simulink model "final_seatmodel_2_version19a"  (R2019a)
settings: Solver=FixedStepAuto  StartTime=0.0  StopTime=50  FixedStep=1  RelTol=1e-3
undefined symbols (not defined in the file or in its folder): F_B_Motion, Head_Rest, Seat_Height, Seat_Recline, Thai_Support
libraries: powerlib_meascontrol x10, simulink x10
settings Model: Creator=A  LastModifiedBy=A

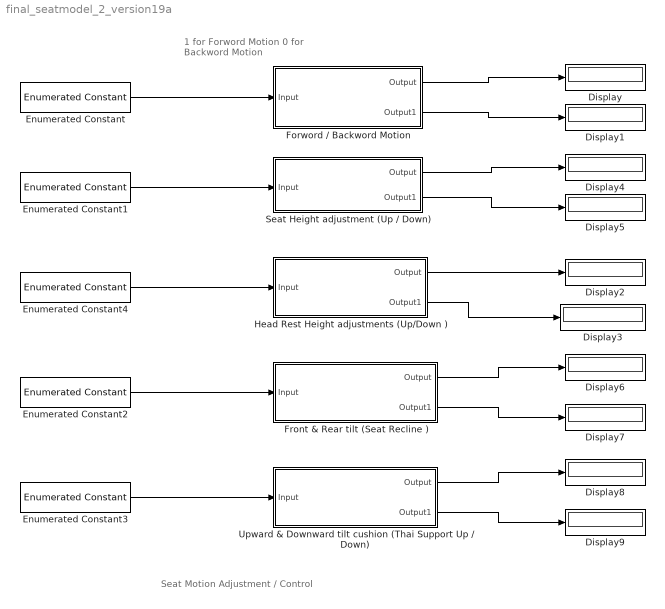
== system final_seatmodel_2_version19a ==
  note: Seat Motion Adjustment / Control
  note: 1 for Forword Motion
      | 0 for Backword Motion
  " Upward & Downward tilt cushion (Thai Support Up / Down) " : Subsystem
  Display{,1..9} (10 alike) : Display
  Enumerated Constant : simulink/Sources/Enumerated Constant  OutDataTypeStr=Enum:F_B_Motion  Value=F_B_Motion.Backword  SampleTime=inf
  Enumerated Constant1 : simulink/Sources/Enumerated Constant  OutDataTypeStr=Enum:Seat_Height  Value=Seat_Height.Down  SampleTime=inf
  Enumerated Constant2 : simulink/Sources/Enumerated Constant  OutDataTypeStr=Enum:Seat_Recline  Value=Seat_Recline.Backword  SampleTime=inf
  Enumerated Constant3 : simulink/Sources/Enumerated Constant  OutDataTypeStr=Enum:Thai_Support  Value=Thai_Support.Down  SampleTime=inf
  Enumerated Constant4 : simulink/Sources/Enumerated Constant  OutDataTypeStr=Enum:Head_Rest  Value=Head_Rest.Down  SampleTime=inf
  Forword / Backword Motion : Subsystem
  "Front & Rear tilt (Seat Recline ) " : Subsystem
  "Head Rest Height adjustments (Up/Down ) " : Subsystem
  "Seat Height adjustment (Up / Down) " : Subsystem
  wires:
  Enumerated Constant3/1 -> " Upward & Downward tilt cushion (Thai Support Up / Down) "/1(Input)
  " Upward & Downward tilt cushion (Thai Support Up / Down) "/1(Output) -> Display8/1
  " Upward & Downward tilt cushion (Thai Support Up / Down) "/2(Output1) -> Display9/1
  Enumerated Constant2/1 -> "Front & Rear tilt (Seat Recline ) "/1(Input)
  "Front & Rear tilt (Seat Recline ) "/1(Output) -> Display6/1
  "Front & Rear tilt (Seat Recline ) "/2(Output1) -> Display7/1
  Enumerated Constant/1 -> Forword / Backword Motion/1(Input)
  Enumerated Constant1/1 -> "Seat Height adjustment (Up / Down) "/1(Input)
  "Seat Height adjustment (Up / Down) "/1(Output) -> Display4/1
  "Seat Height adjustment (Up / Down) "/2(Output1) -> Display5/1
  Enumerated Constant4/1 -> "Head Rest Height adjustments (Up/Down ) "/1(Input)
  "Head Rest Height adjustments (Up/Down ) "/1(Output) -> Display2/1
  "Head Rest Height adjustments (Up/Down ) "/2(Output1) -> Display3/1
  Forword / Backword Motion/2(Output1) -> Display1/1
  Forword / Backword Motion/1(Output) -> Display/1

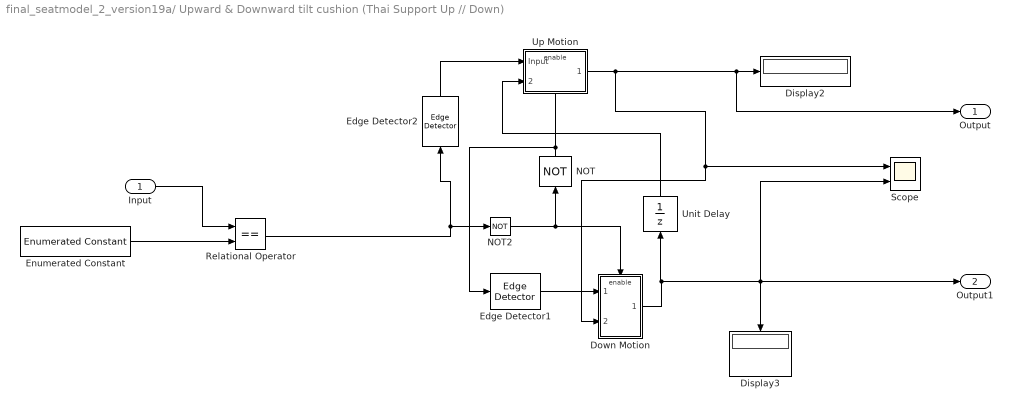
== system final_seatmodel_2_version19a/ Upward & Downward tilt cushion (Thai Support Up // Down)  ==
  Input : Inport
  Display2 : Display
  Display3 : Display
  Down Motion : Subsystem
  Edge Detector1 : powerlib_meascontrol/Logic/Edge Detector  model=Falling  ic=1  Ts=0
      settings: SourceProductBaseCode=PS
  Edge Detector2 : powerlib_meascontrol/Logic/Edge Detector  model=Rising  ic=1  Ts=0
      settings: SourceProductBaseCode=PS
  Enumerated Constant : simulink/Sources/Enumerated Constant  OutDataTypeStr=Enum:Thai_Support  Value=Thai_Support.Up  SampleTime=inf
  NOT : Logic  Operator=NOT  IconShape=distinctive  AllPortsSameDT=off  OutDataTypeStr=boolean
  NOT2 : Logic  Operator=NOT  IconShape=distinctive  AllPortsSameDT=off  OutDataTypeStr=boolean
  Relational Operator : RelationalOperator  Operator===  OutDataTypeStr=boolean  RndMeth=Simplest
  Scope : Scope  NumInputPorts=2
  Unit Delay : UnitDelay  SampleTime=-1  HasFrameUpgradeWarning=on
  Up Motion : Subsystem
  Output : Outport
  Output1 : Outport  Port=2
  wires:
  NOT/1 -> Edge Detector1/1, Up Motion/Enable
  Edge Detector1/1 -> Down Motion/1(Input)
  Down Motion/1(Output) -> Unit Delay/1, Output1/1, Display3/1, Scope/2
  Edge Detector2/1 -> Up Motion/1(Input)
  Relational Operator/1 -> Edge Detector2/1, NOT2/1
  Up Motion/1(Output1) -> Down Motion/2(Input1), Scope/1, Output/1, Display2/1
  Unit Delay/1 -> Up Motion/2(Input1)
  NOT2/1 -> Down Motion/Enable, NOT/1
  Enumerated Constant/1 -> Relational Operator/2
  Input/1 -> Relational Operator/1

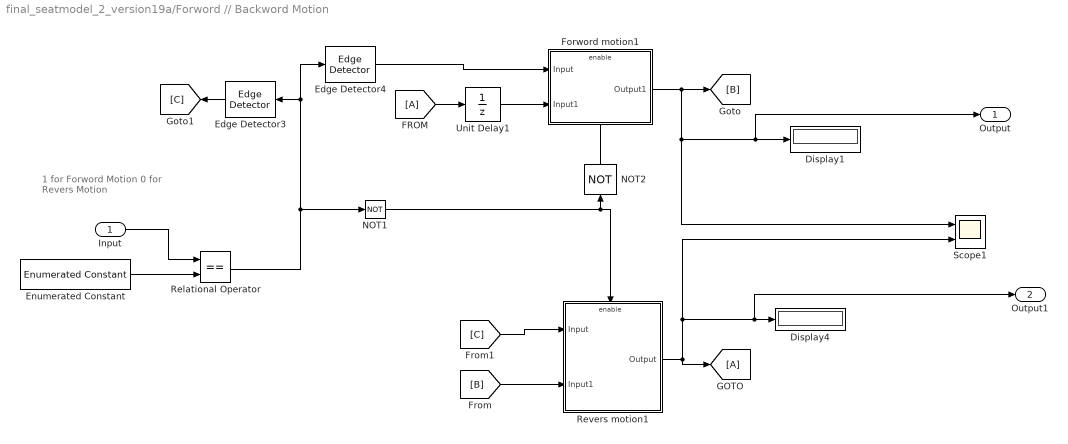
== system final_seatmodel_2_version19a/Forword // Backword Motion ==
  note: 1 for Forword Motion
      | 0 for Revers Motion
  Input : Inport
  Display1 : Display
  Display4 : Display
  Edge Detector3 : powerlib_meascontrol/Logic/Edge Detector  model=Falling  ic=1  Ts=0
      settings: SourceProductBaseCode=PS
  Edge Detector4 : powerlib_meascontrol/Logic/Edge Detector  model=Rising  ic=1  Ts=0
      settings: SourceProductBaseCode=PS
  Enumerated Constant : simulink/Sources/Enumerated Constant  OutDataTypeStr=Enum:F_B_Motion  Value=F_B_Motion.Forword  SampleTime=inf
  Forword motion1 : Subsystem
  NOT1 : Logic  Operator=NOT  IconShape=distinctive  AllPortsSameDT=off  OutDataTypeStr=boolean
  NOT2 : Logic  Operator=NOT  IconShape=distinctive  AllPortsSameDT=off  OutDataTypeStr=boolean
  Relational Operator : RelationalOperator  Operator===  OutDataTypeStr=boolean  RndMeth=Simplest
  Revers motion1 : Subsystem
  Scope1 : Scope  NumInputPorts=2
  Unit Delay1 : UnitDelay  SampleTime=-1  HasFrameUpgradeWarning=on
  Output : Outport
  Output1 : Outport  Port=2
  wires:
  Forword motion1/1(Output1) -> Output/1, Display1/1, Scope1/1, [B]
  Edge Detector3/1 -> [C]
  Revers motion1/1(Output) -> [A], Output1/1, Display4/1, Scope1/2
  Relational Operator/1 -> Edge Detector3/1, Edge Detector4/1, NOT1/1
  NOT2/1 -> Forword motion1/Enable
  [A] -> Unit Delay1/1
  Unit Delay1/1 -> Forword motion1/2(Input1)
  [B] -> Revers motion1/2(Input1)
  Edge Detector4/1 -> Forword motion1/1(Input)
  [C] -> Revers motion1/1(Input)
  NOT1/1 -> Revers motion1/Enable, NOT2/1
  Enumerated Constant/1 -> Relational Operator/2
  Input/1 -> Relational Operator/1

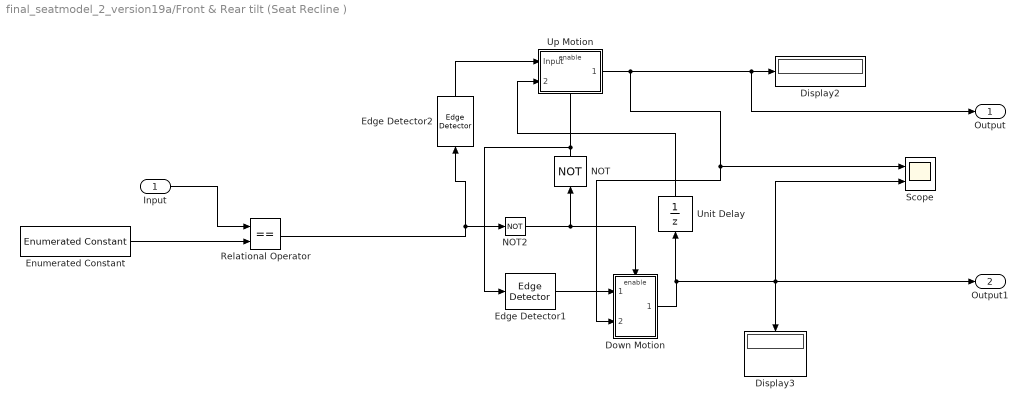
== system final_seatmodel_2_version19a/Front & Rear tilt (Seat Recline )  ==
  Input : Inport
  Display2 : Display
  Display3 : Display
  Down Motion : Subsystem
  Edge Detector1 : powerlib_meascontrol/Logic/Edge Detector  model=Falling  ic=1  Ts=0
      settings: SourceProductBaseCode=PS
  Edge Detector2 : powerlib_meascontrol/Logic/Edge Detector  model=Rising  ic=1  Ts=0
      settings: SourceProductBaseCode=PS
  Enumerated Constant : simulink/Sources/Enumerated Constant  OutDataTypeStr=Enum:Seat_Recline  Value=Seat_Recline.Forword  SampleTime=inf
  NOT : Logic  Operator=NOT  IconShape=distinctive  AllPortsSameDT=off  OutDataTypeStr=boolean
  NOT2 : Logic  Operator=NOT  IconShape=distinctive  AllPortsSameDT=off  OutDataTypeStr=boolean
  Relational Operator : RelationalOperator  Operator===  OutDataTypeStr=boolean  RndMeth=Simplest
  Scope : Scope  NumInputPorts=2
  Unit Delay : UnitDelay  SampleTime=-1  HasFrameUpgradeWarning=on
  Up Motion : Subsystem
  Output : Outport
  Output1 : Outport  Port=2
  wires:
  NOT/1 -> Edge Detector1/1, Up Motion/Enable
  Edge Detector1/1 -> Down Motion/1(Input)
  Down Motion/1(Output) -> Unit Delay/1, Output1/1, Display3/1, Scope/2
  Edge Detector2/1 -> Up Motion/1(Input)
  Relational Operator/1 -> Edge Detector2/1, NOT2/1
  Up Motion/1(Output1) -> Down Motion/2(Input1), Scope/1, Output/1, Display2/1
  Unit Delay/1 -> Up Motion/2(Input1)
  NOT2/1 -> Down Motion/Enable, NOT/1
  Enumerated Constant/1 -> Relational Operator/2
  Input/1 -> Relational Operator/1

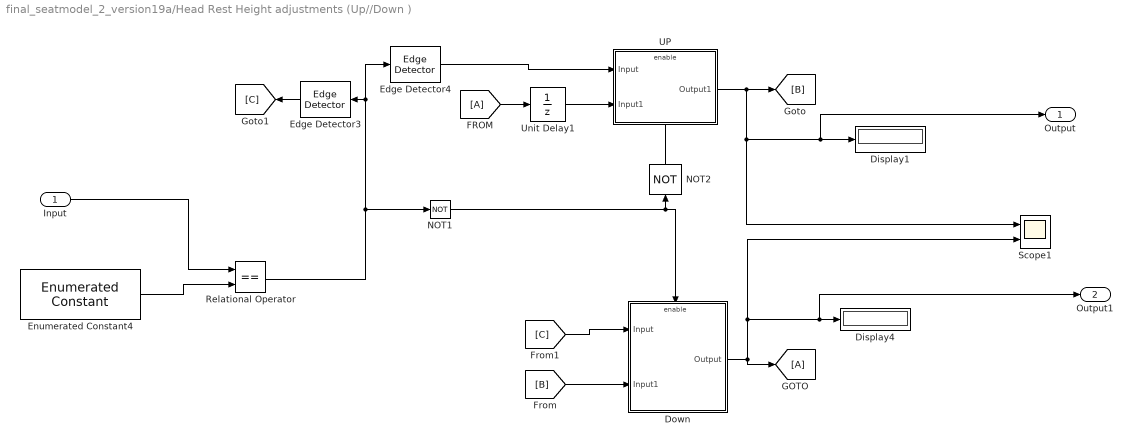
== system final_seatmodel_2_version19a/Head Rest Height adjustments (Up//Down )  ==
  Input : Inport
  Display1 : Display
  Display4 : Display
  Down : Subsystem
  Edge Detector3 : powerlib_meascontrol/Logic/Edge Detector  model=Falling  ic=1  Ts=0
      settings: SourceProductBaseCode=PS
  Edge Detector4 : powerlib_meascontrol/Logic/Edge Detector  model=Rising  ic=1  Ts=0
      settings: SourceProductBaseCode=PS
  Enumerated Constant4 : simulink/Sources/Enumerated Constant  OutDataTypeStr=Enum:Head_Rest  Value=Head_Rest.Up  SampleTime=inf
  NOT1 : Logic  Operator=NOT  IconShape=distinctive  AllPortsSameDT=off  OutDataTypeStr=boolean
  NOT2 : Logic  Operator=NOT  IconShape=distinctive  AllPortsSameDT=off  OutDataTypeStr=boolean
  Relational Operator : RelationalOperator  Operator===  OutDataTypeStr=boolean  RndMeth=Simplest
  Scope1 : Scope  NumInputPorts=2
  UP : Subsystem
  Unit Delay1 : UnitDelay  SampleTime=-1  HasFrameUpgradeWarning=on
  Output : Outport
  Output1 : Outport  Port=2
  wires:
  NOT1/1 -> NOT2/1, Down/Enable
  [C] -> Down/1(Input)
  Edge Detector4/1 -> UP/1(Input)
  [B] -> Down/2(Input1)
  Unit Delay1/1 -> UP/2(Input1)
  [A] -> Unit Delay1/1
  NOT2/1 -> UP/Enable
  Relational Operator/1 -> NOT1/1, Edge Detector4/1, Edge Detector3/1
  Down/1(Output) -> Scope1/2, Display4/1, Output1/1, [A]
  Edge Detector3/1 -> [C]
  UP/1(Output1) -> [B], Scope1/1, Display1/1, Output/1
  Enumerated Constant4/1 -> Relational Operator/2
  Input/1 -> Relational Operator/1

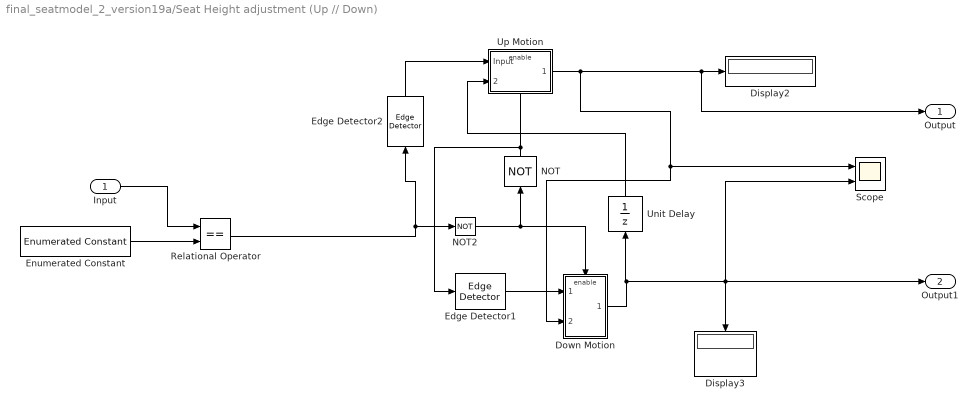
== system final_seatmodel_2_version19a/Seat Height adjustment (Up // Down)  ==
  Input : Inport
  Display2 : Display
  Display3 : Display
  Down Motion : Subsystem
  Edge Detector1 : powerlib_meascontrol/Logic/Edge Detector  model=Falling  ic=1  Ts=0
      settings: SourceProductBaseCode=PS
  Edge Detector2 : powerlib_meascontrol/Logic/Edge Detector  model=Rising  ic=1  Ts=0
      settings: SourceProductBaseCode=PS
  Enumerated Constant : simulink/Sources/Enumerated Constant  OutDataTypeStr=Enum:Seat_Height  Value=Seat_Height.Up  SampleTime=inf
  NOT : Logic  Operator=NOT  IconShape=distinctive  AllPortsSameDT=off  OutDataTypeStr=boolean
  NOT2 : Logic  Operator=NOT  IconShape=distinctive  AllPortsSameDT=off  OutDataTypeStr=boolean
  Relational Operator : RelationalOperator  Operator===  OutDataTypeStr=boolean  RndMeth=Simplest
  Scope : Scope  NumInputPorts=2
  Unit Delay : UnitDelay  SampleTime=-1  HasFrameUpgradeWarning=on
  Up Motion : Subsystem
  Output : Outport
  Output1 : Outport  Port=2
  wires:
  NOT/1 -> Edge Detector1/1, Up Motion/Enable
  Edge Detector1/1 -> Down Motion/1(Input)
  Down Motion/1(Output) -> Unit Delay/1, Output1/1, Display3/1, Scope/2
  Edge Detector2/1 -> Up Motion/1(Input)
  Relational Operator/1 -> Edge Detector2/1, NOT2/1
  Up Motion/1(Output1) -> Down Motion/2(Input1), Scope/1, Output/1, Display2/1
  Unit Delay/1 -> Up Motion/2(Input1)
  NOT2/1 -> Down Motion/Enable, NOT/1
  Enumerated Constant/1 -> Relational Operator/2
  Input/1 -> Relational Operator/1

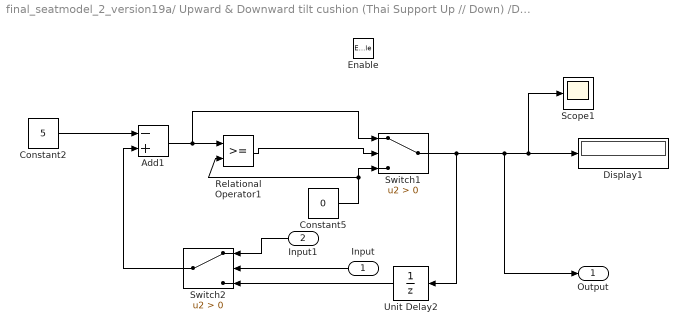
== system final_seatmodel_2_version19a/ Upward & Downward tilt cushion (Thai Support Up // Down) /Down Motion ==
  Input : Inport
  Input1 : Inport  Port=2
  Enable : EnablePort
  Add1 : Sum  Inputs=-+
  Constant2 : Constant  Value=5
  Constant5 : Constant  Value=0
  Display1 : Display
  Relational Operator1 : RelationalOperator  OutDataTypeStr=boolean  RndMeth=Simplest
  Scope1 : Scope
  Switch1 : Switch  Criteria=u2 > Threshold
  Switch2 : Switch  Criteria=u2 > Threshold
  Unit Delay2 : UnitDelay  InitialCondition=100  SampleTime=-1  HasFrameUpgradeWarning=on
  Output : Outport
  wires:
  Relational Operator1/1 -> Switch1/2
  Constant2/1 -> Add1/1
  Add1/1 -> Switch1/1, Relational Operator1/1
  Constant5/1 -> Relational Operator1/2, Switch1/3
  Switch1/1 -> Unit Delay2/1, Output/1, Display1/1, Scope1/1
  Switch2/1 -> Add1/2
  Input1/1 -> Switch2/1
  Unit Delay2/1 -> Switch2/3
  Input/1 -> Switch2/2

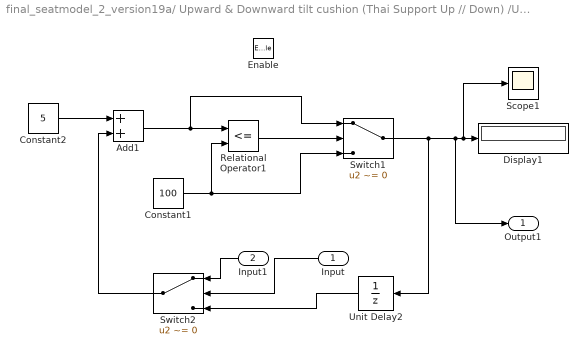
== system final_seatmodel_2_version19a/ Upward & Downward tilt cushion (Thai Support Up // Down) /Up Motion ==
  Input : Inport
  Input1 : Inport  Port=2
  Enable : EnablePort
  Add1 : Sum
  Constant1 : Constant  Value=100
  Constant2 : Constant  Value=5
  Display1 : Display
  Relational Operator1 : RelationalOperator  Operator=<=  OutDataTypeStr=boolean  RndMeth=Simplest
  Scope1 : Scope
  Switch1 : Switch  Criteria=u2 ~= 0
  Switch2 : Switch  Criteria=u2 ~= 0
  Unit Delay2 : UnitDelay  SampleTime=-1  HasFrameUpgradeWarning=on
  Output1 : Outport
  wires:
  Constant1/1 -> Switch1/3, Relational Operator1/2
  Relational Operator1/1 -> Switch1/2
  Constant2/1 -> Add1/1
  Add1/1 -> Switch1/1, Relational Operator1/1
  Switch1/1 -> Unit Delay2/1, Output1/1, Scope1/1, Display1/1
  Input1/1 -> Switch2/1
  Input/1 -> Switch2/2
  Unit Delay2/1 -> Switch2/3
  Switch2/1 -> Add1/2

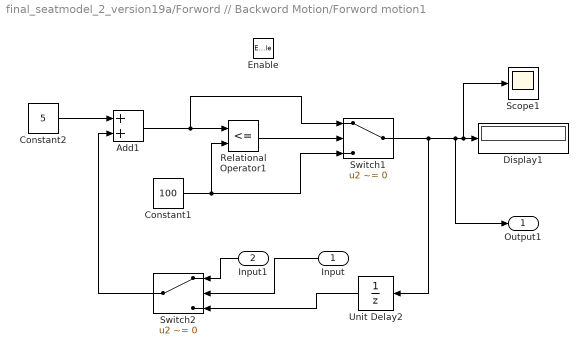
== system final_seatmodel_2_version19a/Forword // Backword Motion/Forword motion1 ==
  Input : Inport
  Input1 : Inport  Port=2
  Enable : EnablePort
  Add1 : Sum
  Constant1 : Constant  Value=100
  Constant2 : Constant  Value=5
  Display1 : Display
  Relational Operator1 : RelationalOperator  Operator=<=  OutDataTypeStr=boolean  RndMeth=Simplest
  Scope1 : Scope
  Switch1 : Switch  Criteria=u2 ~= 0
  Switch2 : Switch  Criteria=u2 ~= 0
  Unit Delay2 : UnitDelay  SampleTime=-1  HasFrameUpgradeWarning=on
  Output1 : Outport
  wires:
  Constant1/1 -> Switch1/3, Relational Operator1/2
  Relational Operator1/1 -> Switch1/2
  Constant2/1 -> Add1/1
  Add1/1 -> Switch1/1, Relational Operator1/1
  Switch1/1 -> Unit Delay2/1, Output1/1, Scope1/1, Display1/1
  Input1/1 -> Switch2/1
  Input/1 -> Switch2/2
  Unit Delay2/1 -> Switch2/3
  Switch2/1 -> Add1/2

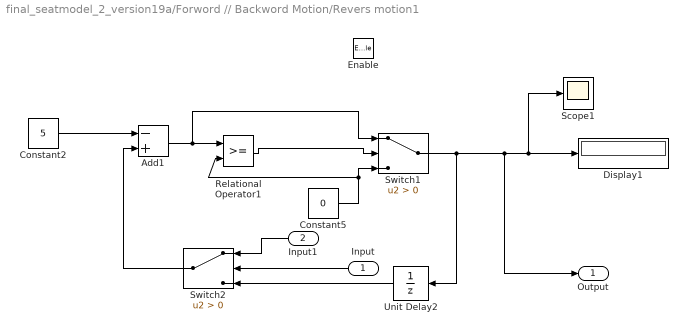
== system final_seatmodel_2_version19a/Forword // Backword Motion/Revers motion1 ==
  Input : Inport
  Input1 : Inport  Port=2
  Enable : EnablePort
  Add1 : Sum  Inputs=-+
  Constant2 : Constant  Value=5
  Constant5 : Constant  Value=0
  Display1 : Display
  Relational Operator1 : RelationalOperator  OutDataTypeStr=boolean  RndMeth=Simplest
  Scope1 : Scope
  Switch1 : Switch  Criteria=u2 > Threshold
  Switch2 : Switch  Criteria=u2 > Threshold
  Unit Delay2 : UnitDelay  InitialCondition=100  SampleTime=-1  HasFrameUpgradeWarning=on
  Output : Outport
  wires:
  Relational Operator1/1 -> Switch1/2
  Constant2/1 -> Add1/1
  Add1/1 -> Switch1/1, Relational Operator1/1
  Constant5/1 -> Relational Operator1/2, Switch1/3
  Switch1/1 -> Unit Delay2/1, Output/1, Display1/1, Scope1/1
  Switch2/1 -> Add1/2
  Input1/1 -> Switch2/1
  Unit Delay2/1 -> Switch2/3
  Input/1 -> Switch2/2

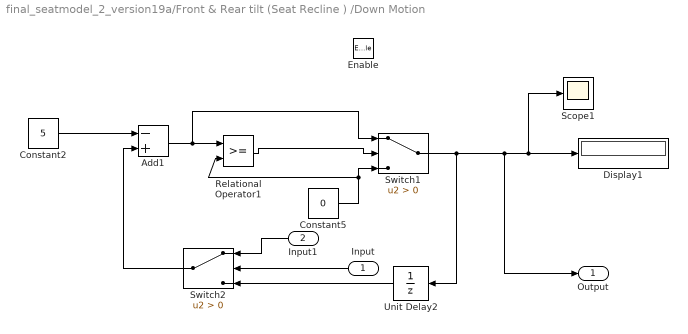
== system final_seatmodel_2_version19a/Front & Rear tilt (Seat Recline ) /Down Motion ==
  Input : Inport
  Input1 : Inport  Port=2
  Enable : EnablePort
  Add1 : Sum  Inputs=-+
  Constant2 : Constant  Value=5
  Constant5 : Constant  Value=0
  Display1 : Display
  Relational Operator1 : RelationalOperator  OutDataTypeStr=boolean  RndMeth=Simplest
  Scope1 : Scope
  Switch1 : Switch  Criteria=u2 > Threshold
  Switch2 : Switch  Criteria=u2 > Threshold
  Unit Delay2 : UnitDelay  InitialCondition=100  SampleTime=-1  HasFrameUpgradeWarning=on
  Output : Outport
  wires:
  Relational Operator1/1 -> Switch1/2
  Constant2/1 -> Add1/1
  Add1/1 -> Switch1/1, Relational Operator1/1
  Constant5/1 -> Relational Operator1/2, Switch1/3
  Switch1/1 -> Unit Delay2/1, Output/1, Display1/1, Scope1/1
  Switch2/1 -> Add1/2
  Input1/1 -> Switch2/1
  Unit Delay2/1 -> Switch2/3
  Input/1 -> Switch2/2

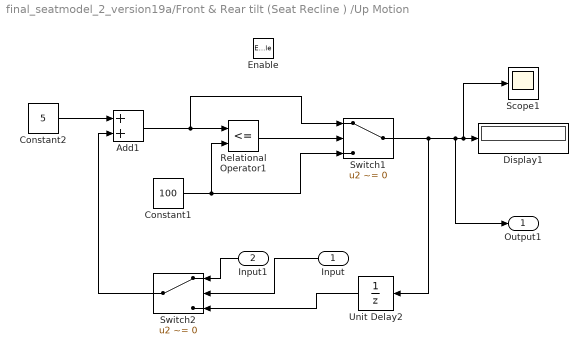
== system final_seatmodel_2_version19a/Front & Rear tilt (Seat Recline ) /Up Motion ==
  Input : Inport
  Input1 : Inport  Port=2
  Enable : EnablePort
  Add1 : Sum
  Constant1 : Constant  Value=100
  Constant2 : Constant  Value=5
  Display1 : Display
  Relational Operator1 : RelationalOperator  Operator=<=  OutDataTypeStr=boolean  RndMeth=Simplest
  Scope1 : Scope
  Switch1 : Switch  Criteria=u2 ~= 0
  Switch2 : Switch  Criteria=u2 ~= 0
  Unit Delay2 : UnitDelay  SampleTime=-1  HasFrameUpgradeWarning=on
  Output1 : Outport
  wires:
  Constant1/1 -> Switch1/3, Relational Operator1/2
  Relational Operator1/1 -> Switch1/2
  Constant2/1 -> Add1/1
  Add1/1 -> Switch1/1, Relational Operator1/1
  Switch1/1 -> Unit Delay2/1, Output1/1, Scope1/1, Display1/1
  Input1/1 -> Switch2/1
  Input/1 -> Switch2/2
  Unit Delay2/1 -> Switch2/3
  Switch2/1 -> Add1/2

== system final_seatmodel_2_version19a/Head Rest Height adjustments (Up//Down ) /Down ==
  Input : Inport
  Input1 : Inport  Port=2
  Enable : EnablePort
  Add1 : Sum  Inputs=-+
  Constant2 : Constant  Value=5
  Constant5 : Constant  Value=0
  Display1 : Display
  Relational Operator1 : RelationalOperator  OutDataTypeStr=boolean  RndMeth=Simplest
  Scope1 : Scope
  Switch1 : Switch  Criteria=u2 > Threshold
  Switch2 : Switch  Criteria=u2 > Threshold
  Unit Delay2 : UnitDelay  InitialCondition=100  SampleTime=-1  HasFrameUpgradeWarning=on
  Output : Outport
  wires:
  Input/1 -> Switch2/2
  Unit Delay2/1 -> Switch2/3
  Input1/1 -> Switch2/1
  Switch2/1 -> Add1/2
  Switch1/1 -> Scope1/1, Display1/1, Output/1, Unit Delay2/1
  Constant5/1 -> Switch1/3, Relational Operator1/2
  Add1/1 -> Relational Operator1/1, Switch1/1
  Constant2/1 -> Add1/1
  Relational Operator1/1 -> Switch1/2

== system final_seatmodel_2_version19a/Head Rest Height adjustments (Up//Down ) /UP ==
  Input : Inport
  Input1 : Inport  Port=2
  Enable : EnablePort
  Add1 : Sum
  Constant1 : Constant  Value=100
  Constant2 : Constant  Value=5
  Display1 : Display
  Relational Operator1 : RelationalOperator  Operator=<=  OutDataTypeStr=boolean  RndMeth=Simplest
  Scope1 : Scope
  Switch1 : Switch  Criteria=u2 ~= 0
  Switch2 : Switch  Criteria=u2 ~= 0
  Unit Delay2 : UnitDelay  SampleTime=-1  HasFrameUpgradeWarning=on
  Output1 : Outport
  wires:
  Switch2/1 -> Add1/2
  Unit Delay2/1 -> Switch2/3
  Input/1 -> Switch2/2
  Input1/1 -> Switch2/1
  Switch1/1 -> Display1/1, Scope1/1, Output1/1, Unit Delay2/1
  Add1/1 -> Relational Operator1/1, Switch1/1
  Constant2/1 -> Add1/1
  Relational Operator1/1 -> Switch1/2
  Constant1/1 -> Relational Operator1/2, Switch1/3

== system final_seatmodel_2_version19a/Seat Height adjustment (Up // Down) /Down Motion ==
  Input : Inport
  Input1 : Inport  Port=2
  Enable : EnablePort
  Add1 : Sum  Inputs=-+
  Constant2 : Constant  Value=5
  Constant5 : Constant  Value=0
  Display1 : Display
  Relational Operator1 : RelationalOperator  OutDataTypeStr=boolean  RndMeth=Simplest
  Scope1 : Scope
  Switch1 : Switch  Criteria=u2 > Threshold
  Switch2 : Switch  Criteria=u2 > Threshold
  Unit Delay2 : UnitDelay  InitialCondition=100  SampleTime=-1  HasFrameUpgradeWarning=on
  Output : Outport
  wires:
  Relational Operator1/1 -> Switch1/2
  Constant2/1 -> Add1/1
  Add1/1 -> Switch1/1, Relational Operator1/1
  Constant5/1 -> Relational Operator1/2, Switch1/3
  Switch1/1 -> Unit Delay2/1, Output/1, Display1/1, Scope1/1
  Switch2/1 -> Add1/2
  Input1/1 -> Switch2/1
  Unit Delay2/1 -> Switch2/3
  Input/1 -> Switch2/2

== system final_seatmodel_2_version19a/Seat Height adjustment (Up // Down) /Up Motion ==
  Input : Inport
  Input1 : Inport  Port=2
  Enable : EnablePort
  Add1 : Sum
  Constant1 : Constant  Value=100
  Constant2 : Constant  Value=5
  Display1 : Display
  Relational Operator1 : RelationalOperator  Operator=<=  OutDataTypeStr=boolean  RndMeth=Simplest
  Scope1 : Scope
  Switch1 : Switch  Criteria=u2 ~= 0
  Switch2 : Switch  Criteria=u2 ~= 0
  Unit Delay2 : UnitDelay  SampleTime=-1  HasFrameUpgradeWarning=on
  Output1 : Outport
  wires:
  Constant1/1 -> Switch1/3, Relational Operator1/2
  Relational Operator1/1 -> Switch1/2
  Constant2/1 -> Add1/1
  Add1/1 -> Switch1/1, Relational Operator1/1
  Switch1/1 -> Unit Delay2/1, Output1/1, Scope1/1, Display1/1
  Input1/1 -> Switch2/1
  Input/1 -> Switch2/2
  Unit Delay2/1 -> Switch2/3
  Switch2/1 -> Add1/2
